simulink model "DesacopladoNL"  (Simulink 7.7)
settings: Solver=ode45  StartTime=0.0  StopTime=2000  RelTol=1e-3
values from neighbouring files (symbols this model uses):
  QT =     [FaseMinima.mat]    (also in FaseNaoMinima.mat; FaseNaoMinimaMudandoApenasGama.mat; settup.m = dynamics())
undefined symbols (not defined in the file or in its folder): get
libraries: simulink x1
settings Model: Creator=Arthur  LastModifiedBy=Arthur
settings DebuggingCC: UnderspecifiedInitializationDetection=Simplified

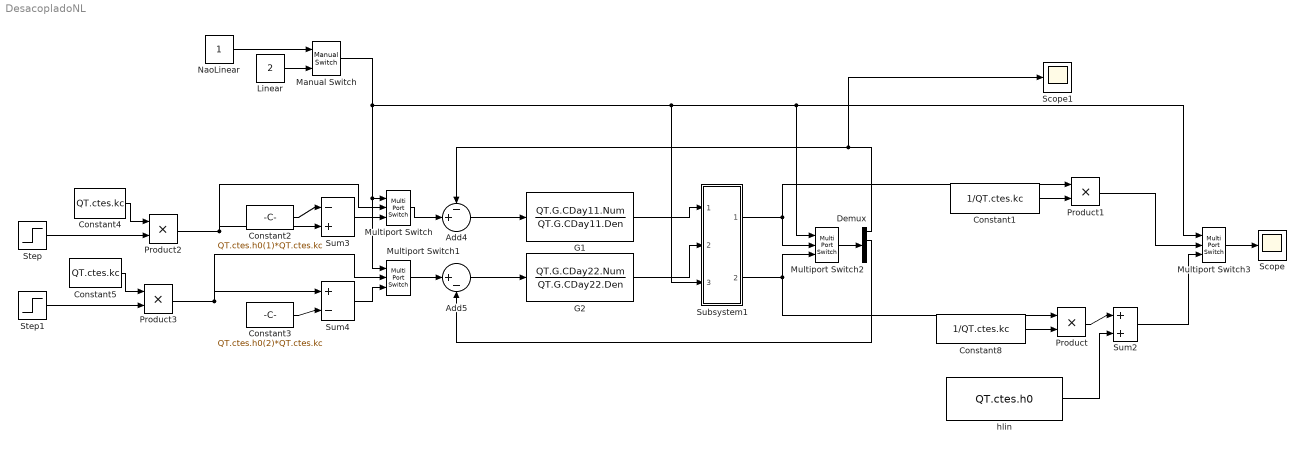
== system DesacopladoNL ==
  Add4 : Sum  Inputs=-+|
  Add5 : Sum  Inputs=|+-
  Constant1 : Constant  Value=1/QT.ctes.kc
  Constant2 : Constant  Value=QT.ctes.h0(1)*QT.ctes.kc
  Constant3 : Constant  Value=QT.ctes.h0(2)*QT.ctes.kc
  Constant4 : Constant  Value=QT.ctes.kc
  Constant5 : Constant  Value=QT.ctes.kc
  Constant8 : Constant  Value=1/QT.ctes.kc
  Demux : Demux
  G1 : TransferFcn  Numerator=QT.G.CDay11.Num  Denominator=QT.G.CDay11.Den
  G2 : TransferFcn  Numerator=QT.G.CDay22.Num  Denominator=QT.G.CDay22.Den
  Linear : Constant  Value=2
  Manual Switch : simulink/Signal Routing/Manual Switch  SystemSampleTime=-1  sw=1  action=0  varsize=off
  Multiport Switch{,1..3} (4 alike) : MultiPortSwitch  Inputs=2  zeroidx=off
  NaoLinear : Constant
  Product{,1..3} (4 alike) : Product  RndMeth=Zero
  Scope : Scope
      settings: TimeRange=2000  YMin=-2e+024  YMax=2.999999999999999e+024
  Scope1 : Scope
      settings: SaveName=ScopeData2
  Step : Step  Time=200  Before=QT.ctes.h0(1)  After=QT.ctes.h0(1)  SampleTime=0
  Step1 : Step  Time=1000  Before=QT.ctes.h0(2)  After=QT.ctes.h0(2)  SampleTime=0
  Subsystem1 : Subsystem
  Sum2 : Sum  Inputs=|++
  Sum3 : Sum  Inputs=|-+
  Sum4 : Sum  Inputs=|+-
  hlin : Constant  Value=QT.ctes.h0
  wires:
  Add5/1 -> G2/1
  Add4/1 -> G1/1
  G2/1 -> Subsystem1/2(In2)
  G1/1 -> Subsystem1/1(In1)
  Subsystem1/2(Out2) -> Product/1, Multiport Switch2/3
  Subsystem1/1(Out1) -> Product1/1, Multiport Switch2/2
  Demux/2 -> Add5/2
  Demux/1 -> Add4/1, Scope1/1
  Multiport Switch2/1 -> Demux/1
  Constant8/1 -> Product/2
  Product/1 -> Sum2/1
  Sum2/1 -> Multiport Switch3/3
  hlin/1 -> Sum2/2
  Constant1/1 -> Product1/2
  Product1/1 -> Multiport Switch3/2
  Constant3/1 -> Sum4/2
  Constant2/1 -> Sum3/1
  Sum4/1 -> Multiport Switch1/3
  Sum3/1 -> Multiport Switch/3
  Multiport Switch/1 -> Add4/2
  Multiport Switch1/1 -> Add5/1
  Manual Switch/1 -> Multiport Switch/1, Multiport Switch1/1, Subsystem1/3(LorNL), Multiport Switch2/1, Multiport Switch3/1
  NaoLinear/1 -> Manual Switch/1
  Linear/1 -> Manual Switch/2
  Multiport Switch3/1 -> Scope/1
  Product2/1 -> Multiport Switch/2, Sum3/2
  Step/1 -> Product2/2
  Constant4/1 -> Product2/1
  Product3/1 -> Multiport Switch1/2, Sum4/1
  Step1/1 -> Product3/2
  Constant5/1 -> Product3/1

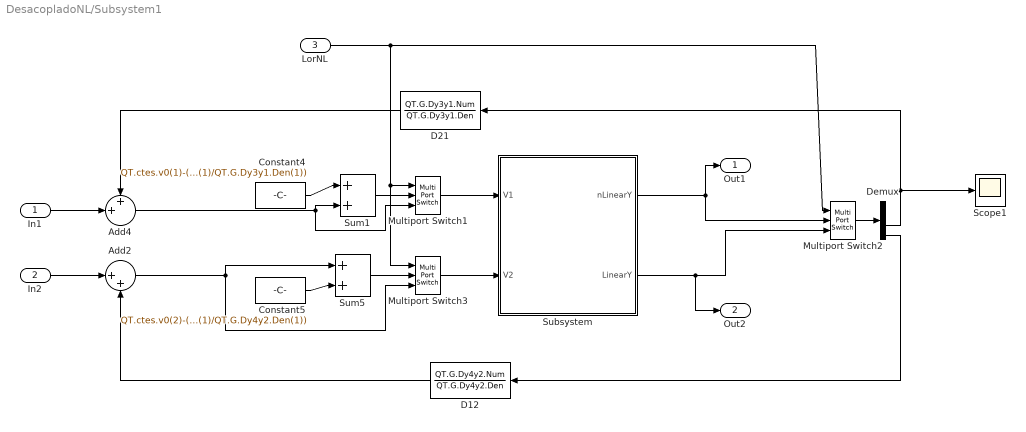
== system DesacopladoNL/Subsystem1 ==
  In1 : Inport
  In2 : Inport  Port=2
  LorNL : Inport  Port=3
  Add2 : Sum  Inputs=|++
  Add4 : Sum  Inputs=++|
  Constant4 : Constant  Value=QT.ctes.v0(1)-(QT.ctes.h0(3)*QT.ctes.kc)*(QT.G.Dy3y1.Num(1)/QT.G.Dy3y1.Den(1))
  Constant5 : Constant  Value=QT.ctes.v0(2)-(QT.ctes.h0(4)*QT.ctes.kc)*(QT.G.Dy4y2.Num(1)/QT.G.Dy4y2.Den(1))
  D12 : TransferFcn  Numerator=QT.G.Dy4y2.Num  Denominator=QT.G.Dy4y2.Den
  D21 : TransferFcn  Numerator=QT.G.Dy3y1.Num  Denominator=QT.G.Dy3y1.Den
  Demux : Demux
  Multiport Switch1 : MultiPortSwitch  Inputs=2  zeroidx=off
  Multiport Switch2 : MultiPortSwitch  Inputs=2  zeroidx=off
  Multiport Switch3 : MultiPortSwitch  Inputs=2  zeroidx=off
  Scope1 : Scope
  Subsystem : Subsystem
  Sum1 : Sum  Inputs=|++
  Sum5 : Sum  Inputs=|++
  Out1 : Outport
  Out2 : Outport  Port=2
  wires:
  D21/1 -> Add4/1
  D12/1 -> Add2/2
  Demux/4 -> D12/1
  Demux/3 -> Scope1/1, D21/1
  Multiport Switch2/1 -> Demux/1
  In1/1 -> Add4/2
  In2/1 -> Add2/1
  Add2/1 -> Sum5/1, Multiport Switch3/3
  Add4/1 -> Sum1/2, Multiport Switch1/3
  Multiport Switch1/1 -> Subsystem/1(V1)
  Multiport Switch3/1 -> Subsystem/2(V2)
  Sum5/1 -> Multiport Switch3/2
  Subsystem/1(nLinearY) -> Out1/1, Multiport Switch2/2
  Subsystem/2(LinearY) -> Out2/1, Multiport Switch2/3
  LorNL/1 -> Multiport Switch2/1, Multiport Switch1/1, Multiport Switch3/1
  Sum1/1 -> Multiport Switch1/2
  Constant4/1 -> Sum1/1
  Constant5/1 -> Sum5/2

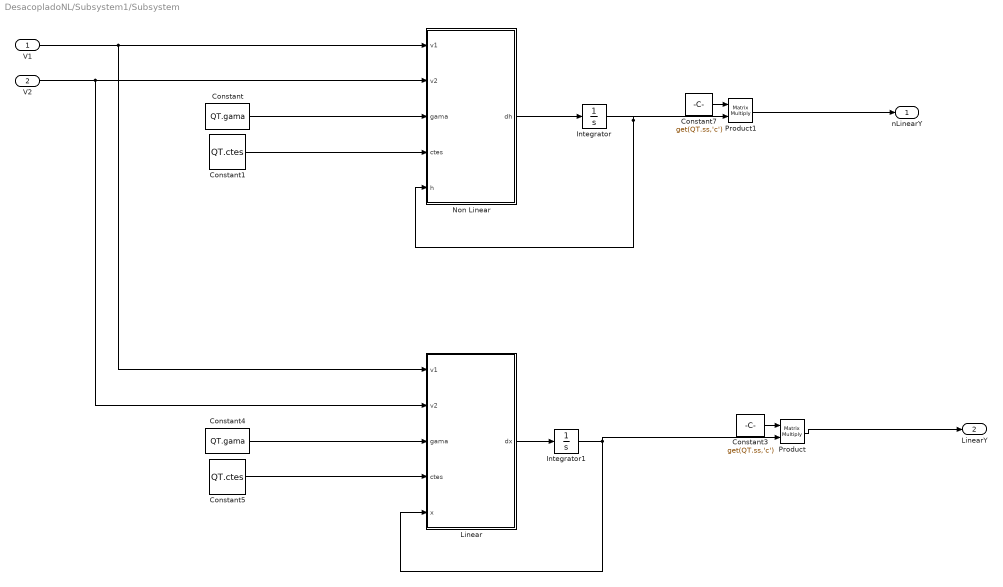
== system DesacopladoNL/Subsystem1/Subsystem ==
  V1 : Inport
  V2 : Inport  Port=2
  Constant : Constant  Value=QT.gama
  Constant1 : Constant  Value=QT.ctes  VectorParams1D=off  OutDataTypeStr=Bus: slBus1
  Constant3 : Constant  Value=get(QT.ss,'c')
  Constant4 : Constant  Value=QT.gama
  Constant5 : Constant  Value=QT.ctes  VectorParams1D=off  OutDataTypeStr=Bus: slBus1
  Constant7 : Constant  Value=get(QT.ss,'c')
  Integrator : Integrator  InitialCondition=QT.ctes.h0
  Integrator1 : Integrator
  Linear : Stateflow chart  TreatAsAtomicUnit=on
  Non Linear : Stateflow chart  TreatAsAtomicUnit=on
  Product : Product  Multiplication=Matrix(*)  RndMeth=Zero
  Product1 : Product  Multiplication=Matrix(*)  RndMeth=Zero
  nLinearY : Outport
  LinearY : Outport  Port=2
  wires:
  Non Linear/1(dh) -> Integrator/1
  Integrator/1 -> Non Linear/5(h), Product1/2
  Constant/1 -> Non Linear/3(gama)
  Constant1/1 -> Non Linear/4(ctes)
  V1/1 -> Linear/1(v1), Non Linear/1(v1)
  V2/1 -> Linear/2(v2), Non Linear/2(v2)
  Linear/1(dx) -> Integrator1/1
  Integrator1/1 -> Linear/5(x), Product/2
  Constant4/1 -> Linear/3(gama)
  Constant5/1 -> Linear/4(ctes)
  Constant3/1 -> Product/1
  Product/1 -> LinearY/1
  Constant7/1 -> Product1/1
  Product1/1 -> nLinearY/1

== matlab function Subsystem1/Subsystem/Linear ==
  data: v1 input double; dx output double; v2 input double; gama input double; ctes input double; x input double
function dx = linsys(v1,v2,gama,ctes,x)
dx = zeros(4,1);    % a column vector
% ----------------

T1=ctes.A1/ctes.a1*sqrt(2*ctes.hlin(1)/ctes.g);
T2=ctes.A2/ctes.a2*sqrt(2*ctes.hlin(2)/ctes.g);
T3=ctes.A3/ctes.a3*sqrt(2*ctes.hlin(3)/ctes.g);
T4=ctes.A4/ctes.a4*sqrt(2*ctes.hlin(4)/ctes.g);

Ass = [-1/T1 0 ctes.A3/(ctes.A1*T3) 0;
    0 -1/T2 0 ctes.A4/(ctes.A2*T4);
    0 0 -1/T3 0;
    0 0 0 -1/T4];
Bss = [gama(1)*ctes.k1/ctes.A1 0;
       0 gama(2)*ctes.k2/ctes.A2;
       0 (1-gama(2))*ctes.k2/ctes.A3;
       (1-gama(1))*ctes.k1/ctes.A4 0];
dx = Ass*x+Bss*[v1;v2];

== matlab function Subsystem1/Subsystem/Non Linear ==
  data: v1 input double; dh output double; v2 input double; gama input double; ctes input double; h input double
function dh = fcn(v1,v2,gama,ctes,h)
dh = zeros(4,1);    % a column vector

    if(h(1)<0)
        h(1)=0;
    end
    if(h(2)<0)
        h(2)=0;
    end
    if(h(3)<0)
        h(3)=0;
    end
    if(h(4)<0)
        h(4)=0;
    end

    
dh(1) = -ctes.a1/ctes.A1*sqrt(2*ctes.g*h(1))+ctes.a3/ctes.A1*sqrt(2*ctes.g*h(3))+gama(1)*ctes.k1*v1/ctes.A1;
dh(2) = -ctes.a2/ctes.A2*sqrt(2*ctes.g*h(2))+ctes.a4/ctes.A2*sqrt(2*ctes.g*h(4))+gama(2)*ctes.k2*v2/ctes.A2;
dh(3) = -ctes.a3/ctes.A3*sqrt(2*ctes.g*h(3))+(1-gama(2))*ctes.k2*v2/ctes.A3; 
dh(4) = -ctes.a4/ctes.A4*sqrt(2*ctes.g*h(4))+(1-gama(1))*ctes.k1*v1/ctes.A4;
